simulink model "flug2d1"  (Simulink 7.0)
settings: Solver=ode45  StartTime=0.0  StopTime=700  RelTol=1e-3
libraries: simulink x2, kalmanlib x2
settings Model: Creator=peter  LastModifiedBy=peter  ExtModeAutoUpdateStatusClock=off

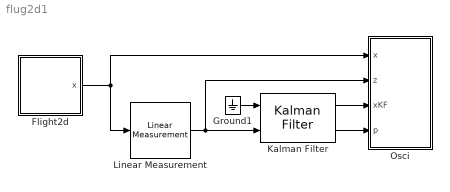
== system flug2d1 ==
  Flight2d : Subsystem  mask(Flight2D){xS=[50;4000], xL=[4500;50], tS=50, tL=70, v0=10, q=0.001, dt=1, seed=17, s=0, tF=0, e=0}
      mask prompts: xS "start point"; xL "landing point"; tS "duration of start"; tL "duration of landing"; v0 "cruise velocity"; q "variance of acceleration"; dt "sample time"; seed "initial seed"; s "total distance"; tF "cruise time"; e "cruise vector"
      mask init:
      | s = norm(xL - xS);
      | tF = (s - v0/2*(tS + tL))/v0;
      | e = (xL - xS)/s;
      mask Display:
      | plot([0.1 0.8], [0.1 0.9])
      | patch(0.1 + 0.05*cos(0:0.2:2*pi), 0.1 + 0.05*sin(0:0.2:2*pi), [1 0 0])
      | patch(0.8 + 0.05*cos(0:0.2:2*pi), 0.9 + 0.05*sin(0:0.2:2*pi), [1 0 0])
      | port_label('output', 1, 'x')
  Ground1 : Ground
  Kalman Filter : kalmanlib/kalman filter/Kalman Filter  SystemSampleTime=-1  A="kron([1, 1, 0.5; 0, 1, 1;  0, 0, 1], [1, 0; 0, 1])"  B=0  H=[0 0 0 0 1 0; 0 0 0 0 0 1]  Q=kron([0.050,0.125,0.167; 0.125,0.333,0.500; 0.167,0.500,1.000],[1, 0; 0, 1])*0.001  R=eye(2)*0.003  x0=[50 4000 0 0 0 0]'  P0=eye(6)*1e-2
  Linear Measurement : kalmanlib/models/Linear Measurement  SystemSampleTime=-1  H=[0 0 0 0 1 0; 0 0 0 0 0 1]  R=eye(2)*0.003  dt=1  seed=[43 44]
  Osci : Subsystem
      settings: OpenFcn=open_system(find_system(gcbh, 'Name', 'Scope'), 'force')
  wires:
  Flight2d/1(x) -> Osci/1(x), Linear Measurement/1
  Linear Measurement/1 -> Kalman Filter/2, Osci/2(z)
  Kalman Filter/2 -> Osci/4(p)
  Kalman Filter/1 -> Osci/3(xKF)
  Ground1/1 -> Kalman Filter/1

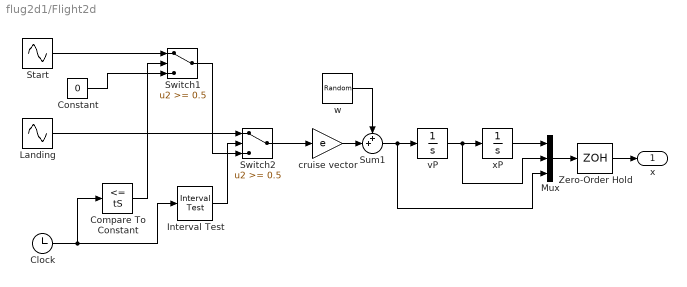
== system flug2d1/Flight2d ==
  Clock : Clock
      settings: Decimation=10
  Compare To Constant : simulink/Logic and Bit Operations/Compare To Constant  SystemSampleTime=-1  relop=<=  const=tS  LogicOutDataTypeMode=boolean  ZeroCross=off
  Constant : Constant  Value=0  OutDataType=sfix(16)  OutScaling=2^0
  Interval Test : simulink/Logic and Bit Operations/Interval Test  SystemSampleTime=-1  IntervalClosedRight=on  uplimit=tS+tF+tL  IntervalClosedLeft=on  lowlimit=tS+tF  LogicOutDataTypeMode=boolean
  Landing : Sin  Amplitude=-v0*pi/(2*tL)  Frequency=pi/tL  Phase=-pi*(tS+tF)/tL  SampleTime=0
  Mux : Mux  Inputs=3
  Start : Sin  Amplitude=v0*pi/(2*tS)  Frequency=pi/tS  SampleTime=0
  Sum1 : Sum  Inputs=++|  OutDataType=sfix(16)  OutScaling=2^0
  Switch1 : Switch  Threshold=0.5
  Switch2 : Switch  Threshold=0.5
  Zero-Order Hold : ZeroOrderHold  SampleTime=dt
  cruise vector : Gain  Gain=e  ParameterDataType=sfix(16)  ParameterScaling=2^0  OutDataType=sfix(16)  OutScaling=2^0
  vP : Integrator  InitialCondition=[0;0]
  w : RandomNumber  Variance=q  Seed=[seed; seed+1]  SampleTime=dt  VectorParams1D=off
  xP : Integrator  InitialCondition=xS
  x : Outport  OutDataType=sfix(16)  OutScaling=2^0
  wires:
  Start/1 -> Switch1/1
  Constant/1 -> Switch1/3
  Compare To Constant/1 -> Switch1/2
  Clock/1 -> Compare To Constant/1, Interval Test/1
  Interval Test/1 -> Switch2/2
  Switch1/1 -> Switch2/3
  Landing/1 -> Switch2/1
  vP/1 -> xP/1, Mux/2
  xP/1 -> Mux/1
  Mux/1 -> Zero-Order Hold/1
  Switch2/1 -> cruise vector/1
  Sum1/1 -> vP/1, Mux/3
  w/1 -> Sum1/1
  Zero-Order Hold/1 -> x/1
  cruise vector/1 -> Sum1/2

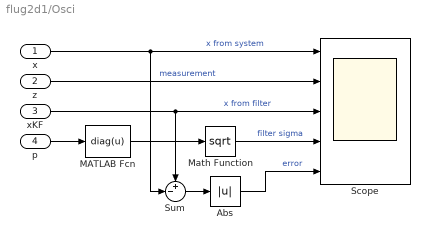
== system flug2d1/Osci ==
  x : Inport  OutDataType=sfix(16)  OutScaling=2^0
  z : Inport  Port=2  OutDataType=sfix(16)  OutScaling=2^0
  xKF : Inport  Port=3  OutDataType=sfix(16)  OutScaling=2^0
  p : Inport  Port=4  OutDataType=sfix(16)  OutScaling=2^0
  Abs : Abs
  MATLAB Fcn : MATLABFcn  MATLABFcn=diag(u)
  Math Function : Math  Operator=sqrt  OutDataType=sfix(16)  OutScaling=2^0  SaturateOnIntegerOverflow=on
  Scope : Scope  NumInputPorts=5
      settings: TimeRange=700  YMin=-1000~-0.5~-1000~0~0  YMax=5000~0.5~5000~600~400
  Sum : Sum  Inputs=+-|  OutDataType=sfix(16)  OutScaling=2^0
  wires:
  p/1 -> MATLAB Fcn/1
  xKF/1 -> Sum/1, Scope/3  "x from filter"
  z/1 -> Scope/2  "measurement"
  x/1 -> Sum/2, Scope/1  "x from system"
  Abs/1 -> Scope/5  "error"
  Sum/1 -> Abs/1
  Math Function/1 -> Scope/4  "filter sigma"
  MATLAB Fcn/1 -> Math Function/1
